simulink library "EVlib"  (R2021a)
settings: Solver=VariableStepAuto  StartTime=0.0  StopTime=10.0  RelTol=1e-3
settings Model: Creator=himi  LastModifiedBy=himi

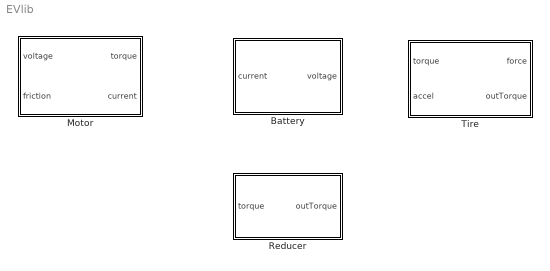
== system EVlib ==
  Battery : Subsystem  mask{SOCinit=100, Rint=0, V0=0, Bcapacity=0}
      mask prompts: SOCinit "Initial SOC [%]"; Rint "Internal Resistance [ohm]"; V0 "Nominal Voltage [V]"; Bcapacity "Battery Capacity"
  Motor : Subsystem  mask{motR=0, motL=0, Km=0}
      mask prompts: motR "Resitance [ohm]"; motL "Inductance [H]"; Km "Torque Coefficient [Nm/A]"
  Reducer : Subsystem  mask{gearRatio=0}
      mask prompts: gearRatio "Gear Ratio"
  Tire : Subsystem  mask{R=0, J=0, tireResistance=0}
      mask prompts: R "Tire Radius [m]"; J "Tire Momentum"; tireResistance "Tire Resistance"

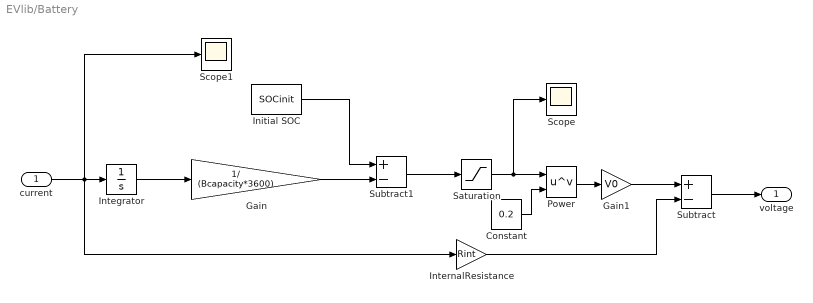
== system EVlib/Battery ==
  current : Inport
  Constant : Constant  Value=0.2
  Gain : Gain  Gain=1/ (Bcapacity*3600)
  Gain1 : Gain  Gain=V0
  Initial SOC : Constant  Value=SOCinit
  Integrator : Integrator
  InternalResistance : Gain  Gain=Rint
  Power : Math  Operator=pow  SaturateOnIntegerOverflow=on
  Saturation : Saturate  UpperLimit=1  LowerLimit=0
  Scope : Scope
  Scope1 : Scope
  Subtract : Sum  Inputs=+-
  Subtract1 : Sum  Inputs=+-
  voltage : Outport
  wires:
  Gain/1 -> Subtract1/2
  Initial SOC/1 -> Subtract1/1
  Subtract1/1 -> Saturation/1
  Gain1/1 -> Subtract/1
  Power/1 -> Gain1/1
  Constant/1 -> Power/2
  Saturation/1 -> Scope/1, Power/1
  InternalResistance/1 -> Subtract/2
  current/1 -> Scope1/1, Integrator/1, InternalResistance/1
  Integrator/1 -> Gain/1
  Subtract/1 -> voltage/1

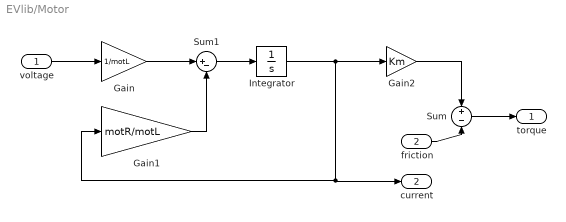
== system EVlib/Motor ==
  voltage : Inport
  friction : Inport  Port=2
  Gain : Gain  Gain=1/motL
  Gain1 : Gain  Gain=motR/motL
  Gain2 : Gain  Gain=Km
  Integrator : Integrator
  Sum : Sum  Inputs=+-
  Sum1 : Sum  Inputs=|+-
  torque : Outport
  current : Outport  Port=2
  wires:
  Gain2/1 -> Sum/1
  friction/1 -> Sum/2
  Sum/1 -> torque/1
  voltage/1 -> Gain/1
  Gain/1 -> Sum1/1
  Sum1/1 -> Integrator/1
  Gain1/1 -> Sum1/2
  Integrator/1 -> current/1, Gain1/1, Gain2/1

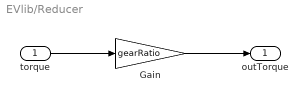
== system EVlib/Reducer ==
  torque : Inport
  Gain : Gain  Gain=gearRatio
  outTorque : Outport
  wires:
  torque/1 -> Gain/1
  Gain/1 -> outTorque/1

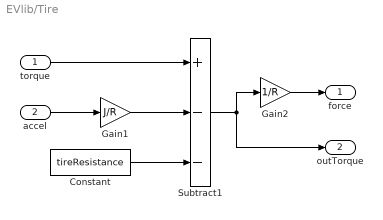
== system EVlib/Tire ==
  torque : Inport
  accel : Inport  Port=2
  Constant : Constant  Value=tireResistance
  Gain1 : Gain  Gain=J/R
  Gain2 : Gain  Gain=1/R
  Subtract1 : Sum  Inputs=+--
  force : Outport
  outTorque : Outport  Port=2
  wires:
  Gain1/1 -> Subtract1/2
  Subtract1/1 -> Gain2/1, outTorque/1
  accel/1 -> Gain1/1
  torque/1 -> Subtract1/1
  Gain2/1 -> force/1
  Constant/1 -> Subtract1/3
